simulink model "Greenhouse"  (R2015a)
settings: Solver=ode45  StartTime=0.0  StopTime=10000.0  RelTol=1e-3
values from neighbouring files (symbols this model uses):
  ac = 0.1    [GreenHouseData.m]
  Av = 2.2    [GreenHouseData.m]
  Ca = 1005    [GreenHouseData.m]
  H = Vol/(len*wid)    [GreenHouseData.m]
  Hin = 35    [GreenHouseData.m]
  Hout = 60    [GreenHouseData.m]
  I = 200    [GreenHouseData.m]
  Kc = 0.028    [GreenHouseData.m]
  Kv = 0.7    [GreenHouseData.m]
  Lc = 0.03    [GreenHouseData.m]
  len = 20    [GreenHouseData.m]
  pa = 1.137    [GreenHouseData.m]
  R = 5    [GreenHouseData.m]
  rv = 0.5    [GreenHouseData.m]
  S = 2*(len*heig+wid*heig)+wid*((wid/2)*tan(angRad))+2*(((wid/2)/cos(angRad))*len)    [GreenHouseData.m]
  Sc = 2*(len*heig+wid*heig)    (= 180)    [GreenHouseData.m]
  tc = 0.85    [GreenHouseData.m]
  Ti = 20    [GreenHouseData.m]
  To = 10    [GreenHouseData.m]
  Vol = len*wid*heig+0.5*wid*((wid/2)*tan(angRad))*len    [GreenHouseData.m]
  Vw = 1    [GreenHouseData.m]
settings Model: Creator=Aakesh Jain  LastModifiedBy=Aakesh Jain

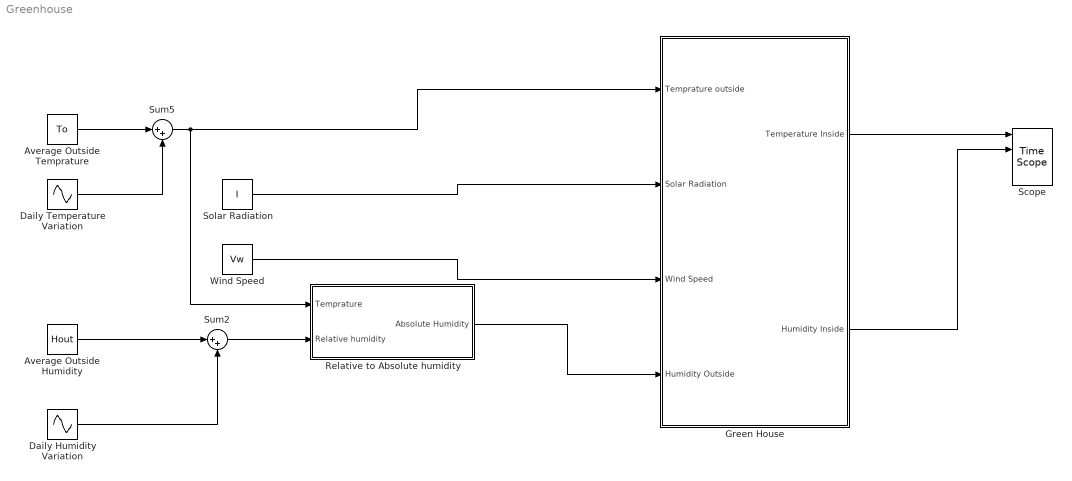
== system Greenhouse ==
  Average Outside Humidity : Constant  Value=Hout
  "Average Outside Temprature " : Constant  Value=To
  Daily Humidity Variation : Sin  Amplitude=5  Frequency=0.005  Phase=1.5708  SampleTime=0
  Daily Temperature Variation : Sin  Amplitude=5  SampleTime=0
  Green House : Subsystem
  Relative to Absolute humidity : Subsystem
  Scope : TimeScope  NumInputPorts=4
  Solar Radiation : Constant  Value=I
  Sum2 : Sum  Inputs=|++
  Sum5 : Sum  Inputs=|++
  Wind Speed : Constant  Value=Vw
  wires:
  "Average Outside Temprature "/1 -> Sum5/1
  Green House/1(Temperature Inside) -> Scope/1
  Sum5/1 -> Relative to Absolute humidity/1(Temprature), Green House/1(Temprature outside)
  Wind Speed/1 -> Green House/3(Wind Speed)
  Relative to Absolute humidity/1(Absolute Humidity) -> Green House/4(Humidity Outside)
  Daily Temperature Variation/1 -> Sum5/2
  Solar Radiation/1 -> Green House/2(Solar Radiation)
  Green House/2(Humidity Inside) -> Scope/2
  Average Outside Humidity/1 -> Sum2/1
  Sum2/1 -> Relative to Absolute humidity/2(Relative humidity)
  Daily Humidity Variation/1 -> Sum2/2

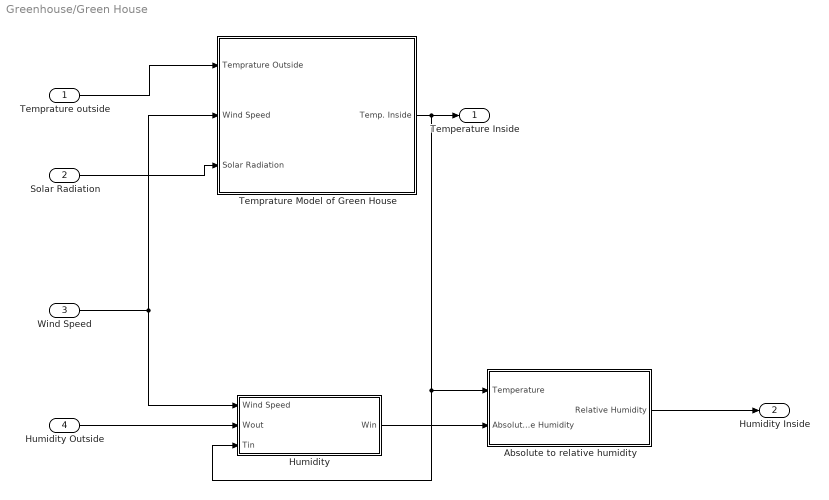
== system Greenhouse/Green House ==
  Temprature outside : Inport
  Solar Radiation : Inport  Port=2
  Wind Speed : Inport  Port=3
  Humidity Outside : Inport  Port=4
  Absolute to relative humidity : Subsystem
  Humidity : Subsystem
  Temprature Model of Green House : Subsystem
  Temperature Inside : Outport
  Humidity Inside : Outport  Port=2
  wires:
  Temprature Model of Green House/1(Temp. Inside) -> Humidity/3("Tin "), Absolute to relative humidity/1(Temperature), Temperature Inside/1
  Wind Speed/1 -> Humidity/1(Wind Speed), Temprature Model of Green House/2(Wind Speed)
  Temprature outside/1 -> Temprature Model of Green House/1(Temprature Outside)
  Solar Radiation/1 -> Temprature Model of Green House/3(Solar Radiation)
  Humidity Outside/1 -> Humidity/2(Wout)
  Humidity/1(Win) -> Absolute to relative humidity/2(Absolute Humidity)
  Absolute to relative humidity/1(Relative Humidity) -> Humidity Inside/1

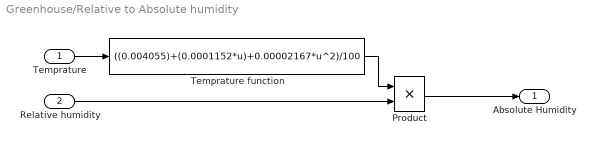
== system Greenhouse/Relative to Absolute humidity ==
  Temprature : Inport
  Relative humidity : Inport  Port=2
  Product : Product
  Temprature function : Fcn  Expr=((0.004055)+(0.0001152*u)+0.00002167*u^2)/100
  Absolute Humidity : Outport
  wires:
  Temprature/1 -> Temprature function/1
  Product/1 -> Absolute Humidity/1
  Relative humidity/1 -> Product/2
  Temprature function/1 -> Product/1

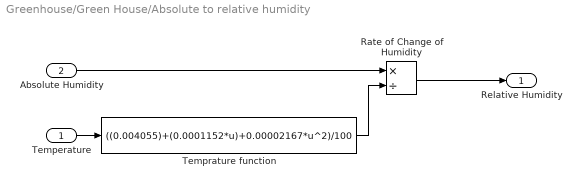
== system Greenhouse/Green House/Absolute to relative humidity ==
  Temperature : Inport
  Absolute Humidity : Inport  Port=2
  Rate of Change of Humidity : Product  Inputs=*/
  Temprature function : Fcn  Expr=((0.004055)+(0.0001152*u)+0.00002167*u^2)/100
  Relative Humidity : Outport
  wires:
  Temprature function/1 -> Rate of Change of Humidity/2
  Absolute Humidity/1 -> Rate of Change of Humidity/1
  Rate of Change of Humidity/1 -> Relative Humidity/1
  Temperature/1 -> Temprature function/1

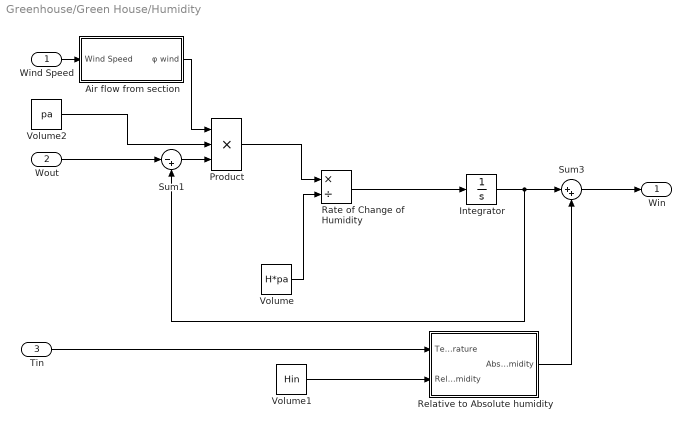
== system Greenhouse/Green House/Humidity ==
  Wind Speed : Inport
  Wout : Inport  Port=2
  "Tin " : Inport  Port=3
  Air flow from section : Subsystem
  Integrator : Integrator
  Product : Product  Inputs=3
  Rate of Change of Humidity : Product  Inputs=*/
  Relative to Absolute humidity : Subsystem
  Sum1 : Sum  Inputs=|-+
  Sum3 : Sum  Inputs=|++
  Volume : Constant  Value=H*pa
  Volume1 : Constant  Value=Hin
  Volume2 : Constant  Value=pa
  Win : Outport
  wires:
  Air flow from section/1(φ wind) -> Product/1
  Sum1/1 -> Product/3
  Volume/1 -> Rate of Change of Humidity/2
  Wout/1 -> Sum1/1
  Wind Speed/1 -> Air flow from section/1(Wind Speed)
  Integrator/1 -> Sum3/1, Sum1/2
  Volume2/1 -> Product/2
  Product/1 -> Rate of Change of Humidity/1
  Rate of Change of Humidity/1 -> Integrator/1
  Sum3/1 -> Win/1
  Relative to Absolute humidity/1(Absolute Humidity) -> Sum3/2
  Volume1/1 -> Relative to Absolute humidity/2(Relative humidity)
  "Tin "/1 -> Relative to Absolute humidity/1(Temprature)

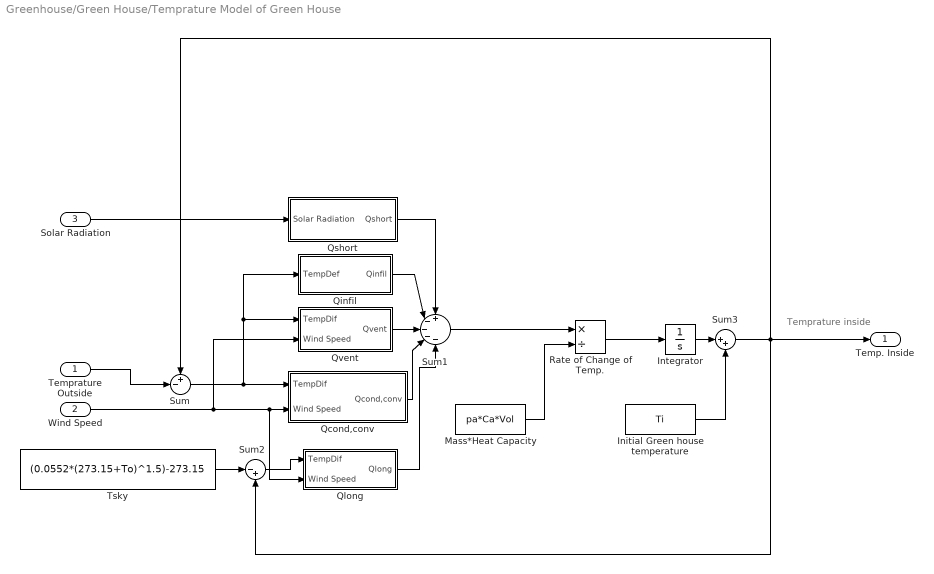
== system Greenhouse/Green House/Temprature Model of Green House ==
  note: Temprature
      | inside
  Temprature Outside : Inport
  Wind Speed : Inport  Port=2
  Solar Radiation : Inport  Port=3
  Initial Green house temperature : Constant  Value=Ti
  Integrator : Integrator
  Mass*Heat Capacity : Constant  Value=pa*Ca*Vol
  Qcond,conv : Subsystem
  Qinfil : Subsystem
  Qlong : Subsystem
  Qshort : Subsystem
  Qvent : Subsystem
  Rate of Change of Temp. : Product  Inputs=*/
  Sum : Sum  Inputs=+-|
  Sum1 : Sum  Inputs=+----
  Sum2 : Sum  Inputs=|-+
  Sum3 : Sum  Inputs=|++
  Tsky : Constant  Value=(0.0552*(273.15+To)^1.5)-273.15
  Temp. Inside : Outport
  wires:
  Sum2/1 -> Qlong/1(TempDif)
  Mass*Heat Capacity/1 -> Rate of Change of Temp./2
  Sum/1 -> Qinfil/1("TempDef "), Qvent/1(TempDif), Qcond,conv/1("TempDif ")
  Qshort/1(Qshort) -> Sum1/1
  Temprature Outside/1 -> Sum/2
  Rate of Change of Temp./1 -> Integrator/1
  Qinfil/1("Qinfil ") -> Sum1/2
  Tsky/1 -> Sum2/1
  Wind Speed/1 -> Qvent/2(Wind Speed), Qlong/2(Wind Speed), Qcond,conv/2(Wind Speed)
  Integrator/1 -> Sum3/1
  Qlong/1(Qlong) -> Sum1/5
  Qcond,conv/1(Qcond,conv) -> Sum1/4
  Solar Radiation/1 -> Qshort/1(Solar Radiation)
  Qvent/1(Qvent) -> Sum1/3
  Sum3/1 -> Sum2/2, Temp. Inside/1, Sum/1
  Initial Green house temperature/1 -> Sum3/2
  Sum1/1 -> Rate of Change of Temp./1

== system Greenhouse/Green House/Humidity/Air flow from section ==
  Wind Speed : Inport
  Product : Product
  Vertical Section : Constant  Value=Av/Sc
  φ wind : Outport
  wires:
  Wind Speed/1 -> Product/1
  Product/1 -> φ wind/1
  Vertical Section/1 -> Product/2

== system Greenhouse/Green House/Humidity/Relative to Absolute humidity ==
  Temprature : Inport
  Relative humidity : Inport  Port=2
  Product : Product
  Temprature function : Fcn  Expr=((0.004055)+(0.0001152*u)+0.00002167*u^2)/100
  Absolute Humidity : Outport
  wires:
  Temprature/1 -> Temprature function/1
  Product/1 -> Absolute Humidity/1
  Relative humidity/1 -> Product/2
  Temprature function/1 -> Product/1

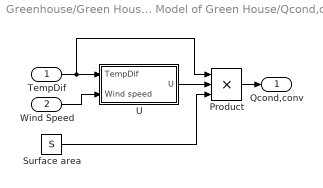
== system Greenhouse/Green House/Temprature Model of Green House/Qcond,conv ==
  "TempDif " : Inport
  Wind Speed : Inport  Port=2
  Product : Product  Inputs=3
  Surface area : Constant  Value=S
  "U " : Subsystem
  Qcond,conv : Outport
  wires:
  Product/1 -> Qcond,conv/1
  "TempDif "/1 -> Product/1, "U "/1("TempDif ")
  Surface area/1 -> Product/3
  "U "/1("U ") -> Product/2
  Wind Speed/1 -> "U "/2(Wind speed)

== system Greenhouse/Green House/Temprature Model of Green House/Qinfil ==
  "TempDef " : Inport
  "Constant " : Constant  Value=pa*Ca*R/3600
  Product : Product
  "Qinfil " : Outport
  wires:
  "Constant "/1 -> Product/1
  Product/1 -> "Qinfil "/1
  "TempDef "/1 -> Product/2

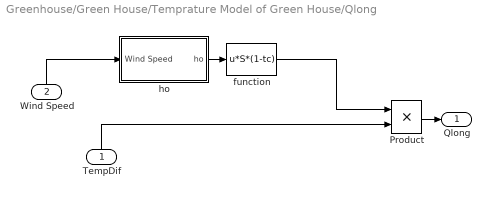
== system Greenhouse/Green House/Temprature Model of Green House/Qlong ==
  TempDif : Inport
  Wind Speed : Inport  Port=2
  " function" : Fcn  Expr=u*S*(1-tc)
  Product : Product
  ho : Subsystem
  Qlong : Outport
  wires:
  TempDif/1 -> Product/2
  " function"/1 -> Product/1
  Product/1 -> Qlong/1
  Wind Speed/1 -> ho/1(Wind Speed)
  ho/1(ho) -> " function"/1

== system Greenhouse/Green House/Temprature Model of Green House/Qshort ==
  Solar Radiation : Inport
  Constant : Constant  Value=ac*tc*S
  Product : Product
  Qshort : Outport
  wires:
  Solar Radiation/1 -> Product/2
  Product/1 -> Qshort/1
  Constant/1 -> Product/1

== system Greenhouse/Green House/Temprature Model of Green House/Qvent ==
  TempDif : Inport
  Wind Speed : Inport  Port=2
  Constant : Constant  Value=rv*Kv*Av*pa*Ca
  Product : Product  Inputs=3
  Qvent : Outport
  wires:
  TempDif/1 -> Product/2
  Wind Speed/1 -> Product/3
  Product/1 -> Qvent/1
  Constant/1 -> Product/1

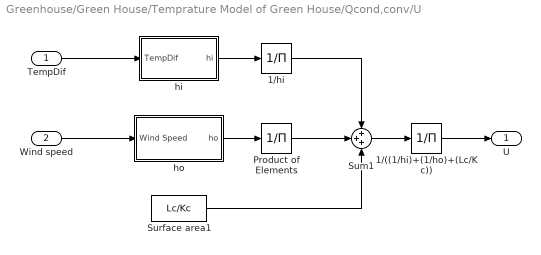
== system Greenhouse/Green House/Temprature Model of Green House/Qcond,conv/U  ==
  "TempDif " : Inport
  Wind speed : Inport  Port=2
  1/((1/hi)+(1/ho)+(Lc/Kc)) : Product  Inputs=/
  1/hi : Product  Inputs=/
  Product of Elements : Product  Inputs=/
  Sum1 : Sum  Inputs=+++
  Surface area1 : Constant  Value=Lc/Kc
  hi : Subsystem
  ho : Subsystem
  "U " : Outport
  wires:
  "TempDif "/1 -> hi/1("TempDif ")
  hi/1("hi ") -> 1/hi/1
  1/((1/hi)+(1/ho)+(Lc/Kc))/1 -> "U "/1
  Sum1/1 -> 1/((1/hi)+(1/ho)+(Lc/Kc))/1
  1/hi/1 -> Sum1/1
  Wind speed/1 -> ho/1(Wind Speed)
  ho/1(ho) -> Product of Elements/1
  Product of Elements/1 -> Sum1/2
  Surface area1/1 -> Sum1/3

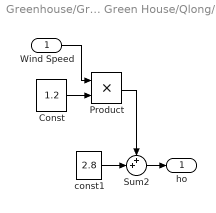
== system Greenhouse/Green House/Temprature Model of Green House/Qlong/ho ==
  Wind Speed : Inport
  Const : Constant  Value=1.2
  Product : Product
  Sum2 : Sum  Inputs=++|
  const1 : Constant  Value=2.8
  ho : Outport
  wires:
  Sum2/1 -> ho/1
  Wind Speed/1 -> Product/1
  Const/1 -> Product/2
  Product/1 -> Sum2/1
  const1/1 -> Sum2/2

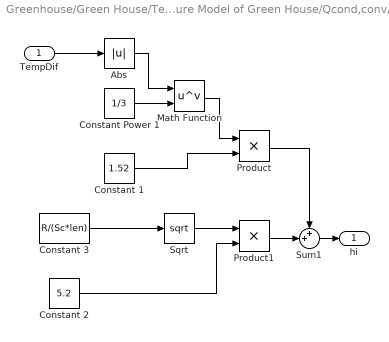
== system Greenhouse/Green House/Temprature Model of Green House/Qcond,conv/U /hi ==
  "TempDif " : Inport
  Abs : Abs
  Constant 1 : Constant  Value=1.52
  Constant 2 : Constant  Value=5.2
  Constant 3 : Constant  Value=R/(Sc*len)
  Constant Power 1 : Constant  Value=1/3
  Math Function : Math  Operator=pow  SaturateOnIntegerOverflow=on
  Product : Product
  Product1 : Product
  Sqrt : Sqrt  SaturateOnIntegerOverflow=on
  Sum1 : Sum  Inputs=++|
  "hi " : Outport
  wires:
  Product1/1 -> Sum1/2
  Constant 2/1 -> Product1/2
  Sum1/1 -> "hi "/1
  Math Function/1 -> Product/1
  Constant Power 1/1 -> Math Function/2
  Product/1 -> Sum1/1
  "TempDif "/1 -> Abs/1
  Constant 1/1 -> Product/2
  Constant 3/1 -> Sqrt/1
  Abs/1 -> Math Function/1
  Sqrt/1 -> Product1/1

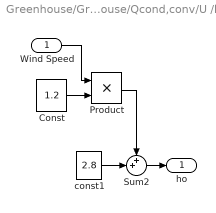
== system Greenhouse/Green House/Temprature Model of Green House/Qcond,conv/U /ho ==
  Wind Speed : Inport
  Const : Constant  Value=1.2
  Product : Product
  Sum2 : Sum  Inputs=++|
  const1 : Constant  Value=2.8
  ho : Outport
  wires:
  Sum2/1 -> ho/1
  Wind Speed/1 -> Product/1
  Const/1 -> Product/2
  Product/1 -> Sum2/1
  const1/1 -> Sum2/2
